simulink model "p2"  (R2021b)
settings: Solver=VariableStepAuto  StartTime=0.0  StopTime=10  RelTol=1e-3
values from neighbouring files (symbols this model uses):
  A = [0 -0.378002311941 0 18.900115597 1 0 0 0 0 7.01473716863 0 -0.379715574203 ... (16 elements, 4x4)]    [Parameters.mat]
  B = [0 -0.0699290719413 0 3.49645359707]    [Parameters.mat]
  cx = [1 0 0 0]    [Parameters.mat]
  k_fast = [18149.2945377 2839.00304412 1519.94169463 86.0344853723]    [Parameters.mat]
  k_slow = [20.7523551145 9.40402411533 21.9918477145 2.35791844149]    [Parameters.mat]
  p_f = 18143.8890275    [Parameters.mat]
  p_s = 15.3468449104    [Parameters.mat]
libraries: simulink x2
settings Model: Creator=hp  LastModifiedBy=hp

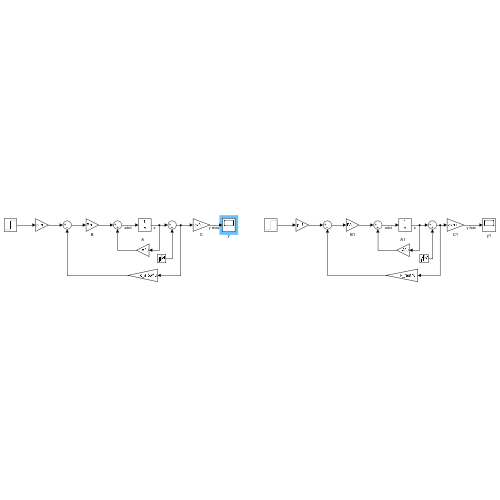
[thumbnail: Simulink's stored preview of the top-level diagram]
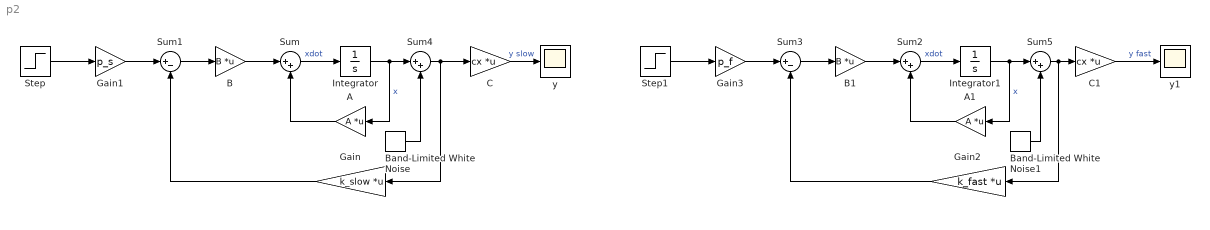
== system p2 ==
  A : Gain  Gain=A  Multiplication=Matrix(K*u)
  A1 : Gain  Gain=A  Multiplication=Matrix(K*u)
  B : Gain  Gain=B  Multiplication=Matrix(K*u)
  B1 : Gain  Gain=B  Multiplication=Matrix(K*u)
  Band-Limited White Noise : simulink/Sources/Band-Limited White Noise  Cov=[0.00002]  Ts=0.5  seed=[23341]
  Band-Limited White Noise1 : simulink/Sources/Band-Limited White Noise  Cov=[0.00002]  Ts=0.5  seed=[23341]
  C : Gain  Gain=cx  Multiplication=Matrix(K*u)
  C1 : Gain  Gain=cx  Multiplication=Matrix(K*u)
  Gain : Gain  Gain=k_slow  Multiplication=Matrix(K*u)
  Gain1 : Gain  Gain=p_s
  Gain2 : Gain  Gain=k_fast  Multiplication=Matrix(K*u)
  Gain3 : Gain  Gain=p_f
  Integrator : Integrator  InitialCondition=[0 0 0 0]
  Integrator1 : Integrator  InitialCondition=[0 0 0 0]
  Step : Step  Time=0  SampleTime=0
  Step1 : Step  Time=0  SampleTime=0
  Sum{,2,4..5} (4 alike) : Sum  Inputs=|++
  Sum1 : Sum  Inputs=|+-
  Sum3 : Sum  Inputs=|+-
  y : Scope
  y1 : Scope
  wires:
  Integrator/1 -> Sum4/1, A/1  "x"
  C/1 -> y/1  "y slow"
  Sum/1 -> Integrator/1  "xdot"
  Gain/1 -> Sum1/2
  Sum1/1 -> B/1
  Gain1/1 -> Sum1/1
  Step/1 -> Gain1/1
  C1/1 -> y1/1  "y fast"
  Sum2/1 -> Integrator1/1  "xdot"
  Gain2/1 -> Sum3/2
  Sum3/1 -> B1/1
  Step1/1 -> Gain3/1
  Gain3/1 -> Sum3/1
  B/1 -> Sum/1
  A/1 -> Sum/2
  Sum4/1 -> Gain/1, C/1
  A1/1 -> Sum2/2
  B1/1 -> Sum2/1
  Integrator1/1 -> Sum5/1, A1/1  "x"
  Sum5/1 -> Gain2/1, C1/1
  Band-Limited White Noise1/1 -> Sum5/2
  Band-Limited White Noise/1 -> Sum4/2
